simulink model "hall_effect_pos_vel_track"  (R2022a)
settings: Solver=FixedStepDiscrete  StartTime=0.0  StopTime=Inf  RelTol=1e-3  EnableMultiTasking=on
undefined symbols (not defined in the file or in its folder): Down, GPTRIP1SEL, GPTRIP2SEL, Hi, High, Impedance, TZ1, TZ2, Up, Z
libraries: c2802xlib x10, c2837xDlib x6, simulink x2, c2000lib x1
settings Model: SimulationMode=external  ExtModeTrigDuration=8  ExtModeArchiveFileName=pep  ExtModeArchiveDirName=C:\Users\adria\Desktop\motor_driver\logs  ExtModeAutoIncOneShot=on  Creator=adria  LastModifiedBy=EEED Stores 381
settings SolverCC: AlgebraicLoopSolver=TrustRegion
settings OptimizationCC: DefaultUnderspecifiedDataType=single  EnhancedBackFolding=on  PassReuseOutputArgsAs=Individual arguments  MaxStackSize=1024  OptimizeBlockOrder=speed  DifferentSizesBufferReuse=on  OptimizationCustomize=off  DenormalBehavior=FlushToZero  EfficientTunableParamExpr=on
settings DebuggingCC: MultiTaskDSMMsg=none  ParameterTunabilityLossMsg=error  UnconnectedInputMsg=warning  UnconnectedOutputMsg=warning  UnconnectedLineMsg=warning  SFMachineParentedDataDiag=warning
settings HardwareCC: ProdBitPerChar=16  ProdBitPerInt=16  ProdBitPerPointer=32  ProdBitPerSizeT=32  ProdBitPerPtrDiffT=32  ProdLargestAtomicInteger=Integer  ProdLargestAtomicFloat=None  ProdWordSize=16  ProdLongLongMode=on  ProdHWDeviceType=Texas Instruments->C2000
settings SFSimCC: MATLABDynamicMemAlloc=off
settings RTWCC: SystemTargetFile=ert.tlc  HardwareBoard=TI Delfino F28379D LaunchPad  TemplateMakefile=ert_default_tmf  Toolchain=Texas Instruments Code Composer Studio (C2000)  DLArmComputeVersion=19.05
settings CodeAppCC: ForceParamTrailComments=on  IgnoreCustomStorageClasses=off  OperatorAnnotations=on  SimulinkDataObjDesc=on  SFDataObjDesc=on  InsertBlockDesc=on
settings ERTTargetCC: CodeReplacementLibrary=TI C28x  ExtMode=on  ExtModeTransport=4  ExtModeStaticAlloc=on  ExtModeStaticAllocSize=10000  ExtModeMexFile=ext_xcp  ExtModeMexArgs='127.0.0.1' 0 17725  ExtModeIntrfLevel=Level2 - Open

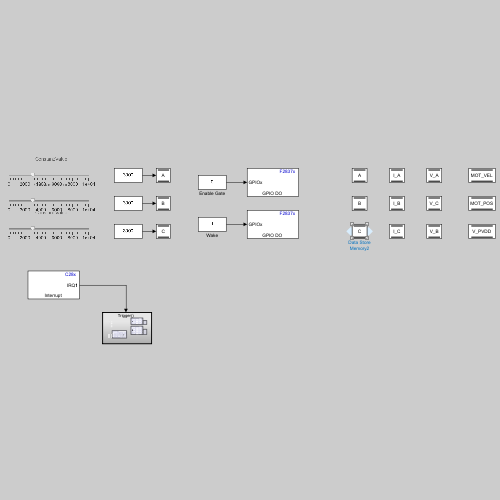
[thumbnail: Simulink's stored preview of the top-level diagram]
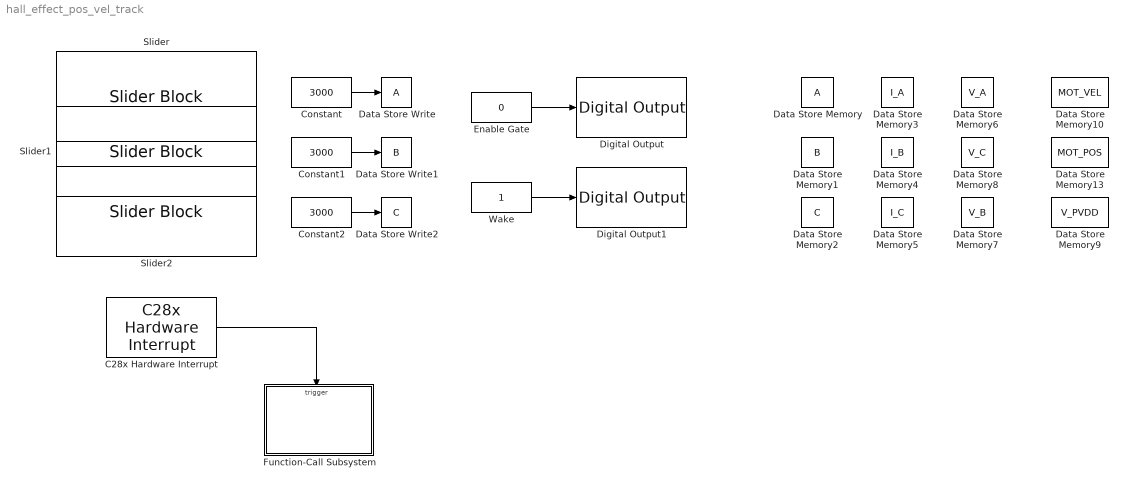
== system hall_effect_pos_vel_track ==
  C28x Hardware Interrupt : c2000lib/Scheduling/C28x Hardware Interrupt  irqnumbers=[1]  pienumbers=[1]  irqpriorities=[30]  irqpreempts=[0]  showinput=off  dspchiptype=C280X
      settings: SourceProductBaseCode=TIC2000
  Constant : Constant  Value=3000  OutDataTypeStr=uint32
  Constant1 : Constant  Value=3000  OutDataTypeStr=uint32
  Constant2 : Constant  Value=3000  OutDataTypeStr=uint32
  Data Store Memory : DataStoreMemory  ReadBeforeWriteMsg=warning  WriteAfterWriteMsg=warning  WriteAfterReadMsg=warning  ShowAdditionalParam=off  OutDataTypeStr=uint32
  Data Store Memory1 : DataStoreMemory  DataStoreName=B  ReadBeforeWriteMsg=warning  WriteAfterWriteMsg=warning  WriteAfterReadMsg=warning  ShowAdditionalParam=off  OutDataTypeStr=uint32
  Data Store Memory10 : DataStoreMemory  DataStoreName=MOT_VEL  ReadBeforeWriteMsg=warning  WriteAfterWriteMsg=warning  WriteAfterReadMsg=warning  ShowAdditionalParam=off  OutDataTypeStr=single
  Data Store Memory13 : DataStoreMemory  DataStoreName=MOT_POS  ReadBeforeWriteMsg=warning  WriteAfterWriteMsg=warning  WriteAfterReadMsg=warning  ShowAdditionalParam=off  OutDataTypeStr=single
  Data Store Memory2 : DataStoreMemory  DataStoreName=C  ReadBeforeWriteMsg=warning  WriteAfterWriteMsg=warning  WriteAfterReadMsg=warning  ShowAdditionalParam=off  OutDataTypeStr=uint32
  Data Store Memory3 : DataStoreMemory  DataStoreName=I_A  ReadBeforeWriteMsg=warning  WriteAfterWriteMsg=warning  WriteAfterReadMsg=warning  ShowAdditionalParam=off  OutDataTypeStr=single
  Data Store Memory4 : DataStoreMemory  DataStoreName=I_B  ReadBeforeWriteMsg=warning  WriteAfterWriteMsg=warning  WriteAfterReadMsg=warning  ShowAdditionalParam=off  OutDataTypeStr=single
  Data Store Memory5 : DataStoreMemory  DataStoreName=I_C  ReadBeforeWriteMsg=warning  WriteAfterWriteMsg=warning  WriteAfterReadMsg=warning  ShowAdditionalParam=off  OutDataTypeStr=single
  Data Store Memory6 : DataStoreMemory  DataStoreName=V_A  ReadBeforeWriteMsg=warning  WriteAfterWriteMsg=warning  WriteAfterReadMsg=warning  ShowAdditionalParam=off  OutDataTypeStr=single
  Data Store Memory7 : DataStoreMemory  DataStoreName=V_B  ReadBeforeWriteMsg=warning  WriteAfterWriteMsg=warning  WriteAfterReadMsg=warning  ShowAdditionalParam=off  OutDataTypeStr=single
  Data Store Memory8 : DataStoreMemory  DataStoreName=V_C  ReadBeforeWriteMsg=warning  WriteAfterWriteMsg=warning  WriteAfterReadMsg=warning  ShowAdditionalParam=off  OutDataTypeStr=single
  Data Store Memory9 : DataStoreMemory  DataStoreName=V_PVDD  ReadBeforeWriteMsg=warning  WriteAfterWriteMsg=warning  WriteAfterReadMsg=warning  ShowAdditionalParam=off  OutDataTypeStr=single
  Data Store Write : DataStoreWrite  IndexOptions=Index vector (dialog)  Indices=1  OutputSizes=1
  Data Store Write1 : DataStoreWrite  DataStoreName=B  IndexOptions=Index vector (dialog)  Indices=1  OutputSizes=1
  Data Store Write2 : DataStoreWrite  DataStoreName=C  IndexOptions=Index vector (dialog)  Indices=1  OutputSizes=1
  Digital Output : c2837xDlib/Digital Output  GPIO_Number=GPIO24~GPIO31  GPIO_Bit0=off  GPIO_BIT0_Toggle=off  GPIO_Bit1=off  GPIO_BIT1_Toggle=off  GPIO_Bit2=on  GPIO_BIT2_Toggle=off  GPIO_Bit3=off  GPIO_BIT3_Toggle=off  GPIO_Bit4=off  GPIO_BIT4_Toggle=off  GPIO_Bit5=off  GPIO_BIT5_Toggle=off  GPIO_Bit6=off  GPIO_BIT6_Toggle=off  GPIO_Bit7=off  GPIO_BIT7_Toggle=off
      settings: SourceProductBaseCode=TIC2000
  Digital Output1 : c2837xDlib/Digital Output  GPIO_Number=GPIO24~GPIO31  GPIO_Bit0=off  GPIO_BIT0_Toggle=off  GPIO_Bit1=off  GPIO_BIT1_Toggle=off  GPIO_Bit2=off  GPIO_BIT2_Toggle=off  GPIO_Bit3=on  GPIO_BIT3_Toggle=off  GPIO_Bit4=off  GPIO_BIT4_Toggle=off  GPIO_Bit5=off  GPIO_BIT5_Toggle=off  GPIO_Bit6=off  GPIO_BIT6_Toggle=off  GPIO_Bit7=off  GPIO_BIT7_Toggle=off
      settings: SourceProductBaseCode=TIC2000
  Enable Gate : Constant  Value=0  OutDataTypeStr=uint32
  Function-Call Subsystem : Subsystem  TreatAsAtomicUnit=on
  Slider : SliderBlock  ScaleMax=10e3
  Slider1 : SliderBlock  ScaleMax=10e3
  Slider2 : SliderBlock  ScaleMax=10e3
  Wake : Constant  OutDataTypeStr=uint32
  wires:
  Enable Gate/1 -> Digital Output/1
  C28x Hardware Interrupt/1 -> Function-Call Subsystem/Trigger
  Constant/1 -> Data Store Write/1
  Constant1/1 -> Data Store Write1/1
  Constant2/1 -> Data Store Write2/1
  Wake/1 -> Digital Output1/1

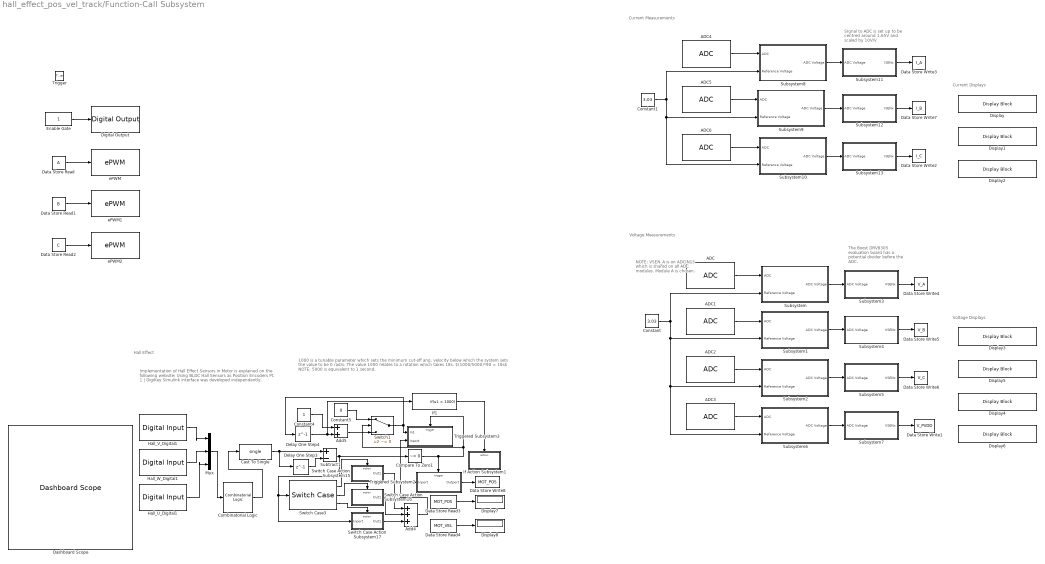
== system hall_effect_pos_vel_track/Function-Call Subsystem ==
  note: Voltage Displays
  note: Current Displays
  note: Current Measurements
  note: Voltage Measurements
  note: NOTE: VSEN_A is on ADCIN15 which is shared on all ADC modules. Module A is chosen.
  note: The Boost DRV8305 evaluation board has a potential divider before the ADC.
  note: SIgnal to ADC is set up to be centred around 1.65V and scaled by 10V/V
  note: 1000 is a tunable parameter which sets the minimum cut-off ang. velocity below which the system sets the value to be 0 rad/s. The value 1000 relates to a rotation which takes 18s.
      | $(1000/5000)*90 = 18s$
      | NOTE: 5000 is equivalent to 1 second.
  note: Hall Effect
  note: Implementation of Hall Effect Sensors in Motor is explained on the following website:
      | Using BLDC Hall Sensors as Position Encoders Pt. 1 | DigiKey
      |
      | Simulink interface was developed independently.
  Trigger : TriggerPort  TriggerType=function-call  VariantControl=Variant  PortDimensions=1
  ADC : c2802xlib/ADC  blkParamProc=C2000_Type4  ADCModule=A  samplingMode=Single sample mode  ADCResolution=12-bit (Single-ended input)  useSOC1=SOC1  useSOC2=SOC0_SOC1  SOCAcquisitionWindow=63  SOCTriggerSource=ePWM4_ADCSOCA  SOCInterruptTrigger=No ADCINT  Ts=-1  dType=uint16  postInterrupt=off  interruptSel=ADCINT2  ADCINTContinuous=off  endma=off  chdma=1  conv1=ADCINA0  conv2=ADCINA0 and ADCINB0  conv1_Type4=ADCIN15  conv2_Type4=ADCIN0 and ADCIN1
      settings: SourceProductName=Embedded Coder Support Package for Texas Instruments C2000 Processors
  ADC1 : c2802xlib/ADC  blkParamProc=C2000_Type4  ADCModule=C  samplingMode=Single sample mode  ADCResolution=12-bit (Single-ended input)  useSOC1=SOC1  useSOC2=SOC0_SOC1  SOCAcquisitionWindow=63  SOCTriggerSource=ePWM4_ADCSOCA  SOCInterruptTrigger=No ADCINT  Ts=-1  dType=uint16  postInterrupt=off  interruptSel=ADCINT1  ADCINTContinuous=off  endma=off  chdma=1  conv1=ADCINA0  conv2=ADCINA0 and ADCINB0  conv1_Type4=ADCIN5  conv2_Type4=ADCIN0 and ADCIN1
      settings: SourceProductName=Embedded Coder Support Package for Texas Instruments C2000 Processors
  ADC2 : c2802xlib/ADC  blkParamProc=C2000_Type4  ADCModule=B  samplingMode=Single sample mode  ADCResolution=12-bit (Single-ended input)  useSOC1=SOC1  useSOC2=SOC0_SOC1  SOCAcquisitionWindow=63  SOCTriggerSource=ePWM4_ADCSOCA  SOCInterruptTrigger=No ADCINT  Ts=-1  dType=uint16  postInterrupt=off  interruptSel=ADCINT1  ADCINTContinuous=off  endma=off  chdma=1  conv1=ADCINA0  conv2=ADCINA0 and ADCINB0  conv1_Type4=ADCIN5  conv2_Type4=ADCIN0 and ADCIN1
      settings: SourceProductName=Embedded Coder Support Package for Texas Instruments C2000 Processors
  ADC3 : c2802xlib/ADC  blkParamProc=C2000_Type4  ADCModule=A  samplingMode=Single sample mode  ADCResolution=12-bit (Single-ended input)  useSOC1=SOC2  useSOC2=SOC0_SOC1  SOCAcquisitionWindow=63  SOCTriggerSource=ePWM4_ADCSOCA  SOCInterruptTrigger=No ADCINT  Ts=-1  dType=uint16  postInterrupt=on  interruptSel=ADCINT1  ADCINTContinuous=off  endma=off  chdma=1  conv1=ADCINA0  conv2=ADCINA0 and ADCINB0  conv1_Type4=ADCIN5  conv2_Type4=ADCIN0 and ADCIN1
      settings: SourceProductName=Embedded Coder Support Package for Texas Instruments C2000 Processors
  ADC4 : c2802xlib/ADC  blkParamProc=C2000_Type4  ADCModule=C  samplingMode=Single sample mode  ADCResolution=12-bit (Single-ended input)  useSOC1=SOC0  useSOC2=SOC0_SOC1  SOCAcquisitionWindow=63  SOCTriggerSource=ePWM4_ADCSOCA  SOCInterruptTrigger=No ADCINT  Ts=-1  dType=uint16  postInterrupt=off  interruptSel=ADCINT2  ADCINTContinuous=off  endma=off  chdma=1  conv1=ADCINA0  conv2=ADCINA0 and ADCINB0  conv1_Type4=ADCIN4  conv2_Type4=ADCIN0 and ADCIN1
      settings: SourceProductName=Embedded Coder Support Package for Texas Instruments C2000 Processors
  ADC5 : c2802xlib/ADC  blkParamProc=C2000_Type4  ADCModule=B  samplingMode=Single sample mode  ADCResolution=12-bit (Single-ended input)  useSOC1=SOC0  useSOC2=SOC0_SOC1  SOCAcquisitionWindow=63  SOCTriggerSource=ePWM4_ADCSOCA  SOCInterruptTrigger=No ADCINT  Ts=-1  dType=uint16  postInterrupt=off  interruptSel=ADCINT2  ADCINTContinuous=off  endma=off  chdma=1  conv1=ADCINA0  conv2=ADCINA0 and ADCINB0  conv1_Type4=ADCIN4  conv2_Type4=ADCIN0 and ADCIN1
      settings: SourceProductName=Embedded Coder Support Package for Texas Instruments C2000 Processors
  ADC6 : c2802xlib/ADC  blkParamProc=C2000_Type4  ADCModule=A  samplingMode=Single sample mode  ADCResolution=12-bit (Single-ended input)  useSOC1=SOC0  useSOC2=SOC0_SOC1  SOCAcquisitionWindow=63  SOCTriggerSource=ePWM4_ADCSOCA  SOCInterruptTrigger=No ADCINT  Ts=-1  dType=uint16  postInterrupt=off  interruptSel=ADCINT1  ADCINTContinuous=on  endma=off  chdma=1  conv1=ADCINA0  conv2=ADCINA0 and ADCINB0  conv1_Type4=ADCIN4  conv2_Type4=ADCIN0 and ADCIN1
      settings: SourceProductName=Embedded Coder Support Package for Texas Instruments C2000 Processors
  Add4 : Sum  Inputs=+++  AccumDataTypeStr=single
  Add5 : Sum
  Cast To Single : DataTypeConversion  OutDataTypeStr=single  SaturateOnIntegerOverflow=off  RndMeth=Floor
  Combinatorial Logic : CombinatorialLogic  TruthTable=[0;1;3;2;5;6;4;7]
  Compare To Zero1 : simulink/Logic and Bit Operations/Compare To Zero  relop=~=  OutDataTypeStr=boolean
  Constant : Constant  Value=3.03  OutDataTypeStr=single
  Constant1 : Constant  Value=3.03  OutDataTypeStr=single
  Constant4 : Constant  OutDataTypeStr=single
  Constant5 : Constant  Value=0  OutDataTypeStr=single
  Dashboard Scope : DashboardScope  TimeSpan=5  Ymin=0  Ymax=7  ScaleAtStop=off
  Data Store Read : DataStoreRead  IndexOptions=Index vector (dialog)  Indices=1  OutputSizes=1
  Data Store Read1 : DataStoreRead  DataStoreName=B  IndexOptions=Index vector (dialog)  Indices=1  OutputSizes=1
  Data Store Read2 : DataStoreRead  DataStoreName=C  IndexOptions=Index vector (dialog)  Indices=1  OutputSizes=1
  Data Store Read3 : DataStoreRead  DataStoreName=MOT_POS  IndexOptions=Index vector (dialog)  Indices=1  OutputSizes=1
  Data Store Read4 : DataStoreRead  DataStoreName=MOT_VEL  IndexOptions=Index vector (dialog)  Indices=1  OutputSizes=1
  Data Store Write1 : DataStoreWrite  DataStoreName=V_PVDD  IndexOptions=Index vector (dialog)  Indices=1  OutputSizes=1
  Data Store Write2 : DataStoreWrite  DataStoreName=I_C  IndexOptions=Index vector (dialog)  Indices=1  OutputSizes=1
  Data Store Write3 : DataStoreWrite  DataStoreName=I_A  IndexOptions=Index vector (dialog)  Indices=1  OutputSizes=1
  Data Store Write4 : DataStoreWrite  DataStoreName=V_A  IndexOptions=Index vector (dialog)  Indices=1  OutputSizes=1
  Data Store Write5 : DataStoreWrite  DataStoreName=V_B  IndexOptions=Index vector (dialog)  Indices=1  OutputSizes=1
  Data Store Write6 : DataStoreWrite  DataStoreName=V_C  IndexOptions=Index vector (dialog)  Indices=1  OutputSizes=1
  Data Store Write7 : DataStoreWrite  DataStoreName=I_B  IndexOptions=Index vector (dialog)  Indices=1  OutputSizes=1
  Data Store Write8 : DataStoreWrite  DataStoreName=MOT_POS  IndexOptions=Index vector (dialog)  Indices=1  OutputSizes=1
  Delay One Step3 : Delay  DelayLength=1
  Delay One Step4 : Delay  DelayLength=1
  Digital Output : c2837xDlib/Digital Output  GPIO_Number=GPIO48~GPIO55  GPIO_Bit0=off  GPIO_BIT0_Toggle=off  GPIO_Bit1=off  GPIO_BIT1_Toggle=off  GPIO_Bit2=off  GPIO_BIT2_Toggle=off  GPIO_Bit3=off  GPIO_BIT3_Toggle=off  GPIO_Bit4=on  GPIO_BIT4_Toggle=on  GPIO_Bit5=off  GPIO_BIT5_Toggle=off  GPIO_Bit6=off  GPIO_BIT6_Toggle=off  GPIO_Bit7=off  GPIO_BIT7_Toggle=off
      settings: SourceProductBaseCode=TIC2000
  Display{,1..6} (7 alike) : DisplayBlock  LabelPosition=Hide  Transparency=1
  Display7 : Display
  Display8 : Display
  Enable Gate : Constant  OutDataTypeStr=uint32
  Hall_U_Digital1 : c2837xDlib/Digital Input  GPIO_Number=GPIO120~GPIO127  GPIO_Bit0=off  GPIO_Bit1=off  GPIO_Bit2=off  GPIO_Bit3=off  GPIO_Bit4=on  GPIO_Bit5=off  GPIO_Bit6=off  GPIO_Bit7=off  sampleTime=-1  dataType=auto  GPIO_Bit0_Qualification=Sync to SYSCLKOUT  GPIO_Bit1_Qualification=Sync to SYSCLKOUT  GPIO_Bit2_Qualification=Sync to SYSCLKOUT  GPIO_Bit3_Qualification=Sync to SYSCLKOUT  GPIO_Bit4_Qualification=Sync to SYSCLKOUT  GPIO_Bit5_Qualification=Sync to SYSCLKOUT  GPIO_Bit6_Qualification=Sync to SYSCLKOUT  GPIO_Bit7_Qualification=Sync to SYSCLKOUT  Qualification_Period=-1
      settings: SourceProductBaseCode=TIC2000
  Hall_V_Digital1 : c2837xDlib/Digital Input  GPIO_Number=GPIO24~GPIO31  GPIO_Bit0=off  GPIO_Bit1=off  GPIO_Bit2=off  GPIO_Bit3=off  GPIO_Bit4=off  GPIO_Bit5=on  GPIO_Bit6=off  GPIO_Bit7=off  sampleTime=-1  dataType=auto  GPIO_Bit0_Qualification=Sync to SYSCLKOUT  GPIO_Bit1_Qualification=Sync to SYSCLKOUT  GPIO_Bit2_Qualification=Sync to SYSCLKOUT  GPIO_Bit3_Qualification=Sync to SYSCLKOUT  GPIO_Bit4_Qualification=Sync to SYSCLKOUT  GPIO_Bit5_Qualification=Sync to SYSCLKOUT  GPIO_Bit6_Qualification=Sync to SYSCLKOUT  GPIO_Bit7_Qualification=Sync to SYSCLKOUT  Qualification_Period=-1
      settings: SourceProductBaseCode=TIC2000
  Hall_W_Digital1 : c2837xDlib/Digital Input  GPIO_Number=GPIO120~GPIO127  GPIO_Bit0=off  GPIO_Bit1=off  GPIO_Bit2=off  GPIO_Bit3=off  GPIO_Bit4=off  GPIO_Bit5=on  GPIO_Bit6=off  GPIO_Bit7=off  sampleTime=-1  dataType=auto  GPIO_Bit0_Qualification=Sync to SYSCLKOUT  GPIO_Bit1_Qualification=Sync to SYSCLKOUT  GPIO_Bit2_Qualification=Sync to SYSCLKOUT  GPIO_Bit3_Qualification=Sync to SYSCLKOUT  GPIO_Bit4_Qualification=Sync to SYSCLKOUT  GPIO_Bit5_Qualification=Sync to SYSCLKOUT  GPIO_Bit6_Qualification=Sync to SYSCLKOUT  GPIO_Bit7_Qualification=Sync to SYSCLKOUT  Qualification_Period=-1
      settings: SourceProductBaseCode=TIC2000
  If Action Subsystem1 : Subsystem  TreatAsAtomicUnit=on
  If1 : If  IfExpression=u1 > 1000  ShowElse=off
  Mux : Mux  Inputs=3
  Subsystem : Subsystem
  Subsystem1 : Subsystem
  Subsystem10 : Subsystem
  Subsystem11 : Subsystem
  Subsystem12 : Subsystem
  Subsystem13 : Subsystem
  Subsystem2 : Subsystem
  Subsystem3 : Subsystem
  Subsystem4 : Subsystem
  Subsystem5 : Subsystem
  Subsystem6 : Subsystem
  Subsystem7 : Subsystem
  Subsystem8 : Subsystem
  Subsystem9 : Subsystem
  Subtract1 : Sum  Inputs=+-
  Switch Case Action Subsystem15 : Subsystem  TreatAsAtomicUnit=on
  Switch Case Action Subsystem16 : Subsystem  TreatAsAtomicUnit=on
  Switch Case Action Subsystem17 : Subsystem  TreatAsAtomicUnit=on
  Switch Case3 : SwitchCase  CaseConditions={-5,5}
  Switch1 : Switch  Criteria=u2 ~= 0  SaturateOnIntegerOverflow=off  InputSameDT=off
  Triggered Subsystem2 : Subsystem  TreatAsAtomicUnit=on
  Triggered Subsystem3 : Subsystem  TreatAsAtomicUnit=on
  ePWM : c2802xlib/ePWM  PwmType=C2000_Type4  useModule=ePWM4  ePWMxLINKTBPRD=Not Linked  periodUnits=Seconds  timerSource=Specify via dialog  timerPeriod_clk=64000  timerPeriod_sec=1/10e3  tbshadow=Counter equals to zero  countingMode=Up-Down  phaseActiveEnable=Disable  phaseDirection=Count down after sync  phaseActive=0  synchronizationEnable=off  dcaevt1Sync=off  dcbevt1Sync=off  synchronizationOption=Counter equals to zero (CTR=Zero)  perSynchronizationOption=Counter equals to period (CTR=PRD)  clockPrescale=1  HSclockPrescale=1  enswap=off  ePWMxAStatus=on  ePWMxAactionLogic1=Set  ePWMxAactionLogic2=Clear  ePWMxAactionLogic3=Clear  ePWMxAactionLogic4=Set  ePWMxAactionLogic5=Do nothing  ePWMxAactionLogic6=Do nothing  ePWMxACSFenable=off  ePWMxACSFvalue=Forcing disable  ePWMxASFreload=Zero  ePWMxBStatus=on  ePWMxBactionLogic1=Clear  ePWMxBactionLogic2=Set  ePWMxBactionLogic3=Set  ePWMxBactionLogic4=Clear  ePWMxBactionLogic5=Do nothing  ePWMxBactionLogic6=Do nothing  ePWMxBCSFenable=off  ePWMxBCSFvalue=Forcing disable  ePWMxBSFreload=Zero  ePWNxBOutWay=off  ePWMxLINKCMPA=Not Linked  CMPAUnits=Clock cycles  CMPASource=Input port  CMPAValue_per=50  CMPAValue_clk=32000  enCMPAshadow=Counter equals to zero (CTR=Zero)  ePWMxLINKCMPB=Not Linked  CMPBUnits=Clock cycles  CMPBSource=Specify via dialog  CMPBValue_per=50  CMPBValue_clk=32000  enCMPBshadow=Counter equals to zero (CTR=Zero)  ePWMxLINKCMPC=Not Linked  CMPCUnits=Clock cycles  CMPCSource=Specify via dialog  CMPCValue_per=50  CMPCValue_clk=32000  enCMPCshadow=Counter equals to zero (CTR=Zero)  ePWMxLINKCMPD=Not Linked  CMPDUnits=Clock cycles  CMPDSource=Specify via dialog  CMPDValue_per=50  CMPDValue_clk=32000  enCMPDshadow=Counter equals to zero (CTR=Zero)  enableDBePWMxA=on  enableDBePWMxB=on  enhalfcycle=off  DBpolarity=Active high complementary (AHC)  DBedgeDelay=Positive  DBSource_ePWMxA=ePWMxA  DBSource_ePWMxB=ePWMxA  DBPeriodUnits=Clock cycles  DBperiodSource=Specify via dialog  REDperiod=10  FEDperiod=10  REDperiod_sec=0  FEDperiod_sec=0  LoadModeDBRED=Immediate without using shadow  LoadModeDBFED=Immediate without using shadow  adcstartModuleA=on  adcrequestEventA=First event  adcstartEventA=Digital Compare Module A Event 1 start of conversion (DCAEVT1.soc)  adcstartEventA_type2=Counter equals to zero (CTR=Zero)  adcstartModuleB=off  adcrequestEventB=First event  adcstartEventB=Counter equals to zero (CTR=Zero)  adcstartEventB_type2=Counter equals to zero (CTR=Zero)  intEn=off  intPrd=First event  intSel=Counter equals to zero (CTR=Zero)  intSel_type2=Counter equals to zero (CTR=Zero)  hrpe=off  enHRPWM=off  HRPWM_LoadMode=Counter equals to period (CTR=PRD)  HRPWM_CTLMode=Duty or Period control mode  HRPWM_EDGMode=Both edge  hrpeb=off  enHRPWMB=off  HRPWM_LoadModeB=Counter equals to zero (CTR=ZERO)  HRPWM_CTLModeB=Duty or Period control mode  HRPWM_EDGModeB=Both edge  enHRDBRED=off  enHRDBFED=off  enSFO=on  enautoconv=on  chopperEnable=off  chopperFrequency=1  chopperFirstwidth=1  chopperDuty=12.5%  tripZonesource=Specify via dialog  tzselOSHT1=off  tzselOSHT2=off  tzselOSHT3=off  tzselOSHDCAEV1=off  tzselOSHDCBEV1=off  tzselCBC1=off  tzselCBC2=off  tzselCBC3=off  tzselCBCDCAEV2=off  tzselCBCDCBEV2=off  tzselOSHT4=off  tzselOSHT5=off  tzselOSHT6=off  tzselCBC4=off  tzselCBC5=off  tzselCBC6=off  enTzOstIntr=off  enTzCbcIntr=off  enTzDCAEVT1Intr=off  enTzDCAEVT2Intr=off  enTzDCBEVT1Intr=off  enTzDCBEVT2Intr=off  ePWMxAforced=Hi-Z(High-Impedance)  ePWMxBforced=Hi-Z(High-Impedance)  DCAEVT1forced=No action  DCBEVT1forced=No action  DCAEVT2forced=No action  DCBEVT2forced=No action  dcah=Trip Zone 1 input (TZ1)  dcal=Trip Zone 2 input (TZ2)  dcbh=Trip Zone 1 input (TZ1)  dcbl=Trip Zone 2 input (TZ2)  dcah_type2=GPTRIP1SEL/(TZ1)  dcal_type2=GPTRIP2SEL/(TZ2)  dcbh_type2=GPTRIP1SEL/(TZ1)  dcbl_type2=GPTRIP2SEL/(TZ2)  gendcaevt1=Event disabled  gendcaevt2=Event disabled  gendcbevt1=Event disabled  gendcbevt2=Event disabled  dcaevt1src=DCAEVT1 with sync  dcaevt2src=DCAEVT2 with sync  dcbevt1src=DCBEVT1 with sync  dcbevt2src=DCBEVT2 with sync  pulsesel=Counter equals to zero (CTR=Zero)  blankinv=off  blankoffset=0  blankwidth=0  evsrcsel=Filtered version of DCAEVT1 (DCAEVT1FILT)  encape=off
      settings: SourceProductName=Embedded Coder Support Package for Texas Instruments C2000 Processors
  ePWM1 : c2802xlib/ePWM  PwmType=C2000_Type4  useModule=ePWM5  ePWMxLINKTBPRD=Not Linked  periodUnits=Seconds  timerSource=Specify via dialog  timerPeriod_clk=64000  timerPeriod_sec=1/10e3  tbshadow=Counter equals to zero  countingMode=Up-Down  phaseActiveEnable=Set counter to phase value specified via dialog  phaseDirection=Count down after sync  phaseActive=0  synchronizationEnable=off  dcaevt1Sync=off  dcbevt1Sync=off  synchronizationOption=Pass through (EPWMxSYNCI or SWFSYNC)  perSynchronizationOption=Counter equals to period (CTR=PRD)  clockPrescale=1  HSclockPrescale=1  enswap=off  ePWMxAStatus=on  ePWMxAactionLogic1=Set  ePWMxAactionLogic2=Clear  ePWMxAactionLogic3=Clear  ePWMxAactionLogic4=Set  ePWMxAactionLogic5=Do nothing  ePWMxAactionLogic6=Do nothing  ePWMxACSFenable=off  ePWMxACSFvalue=Forcing disable  ePWMxASFreload=Zero  ePWMxBStatus=on  ePWMxBactionLogic1=Clear  ePWMxBactionLogic2=Set  ePWMxBactionLogic3=Set  ePWMxBactionLogic4=Clear  ePWMxBactionLogic5=Do nothing  ePWMxBactionLogic6=Do nothing  ePWMxBCSFenable=off  ePWMxBCSFvalue=Forcing disable  ePWMxBSFreload=Zero  ePWNxBOutWay=off  ePWMxLINKCMPA=Not Linked  CMPAUnits=Clock cycles  CMPASource=Input port  CMPAValue_per=50  CMPAValue_clk=32000  enCMPAshadow=Counter equals to zero (CTR=Zero)  ePWMxLINKCMPB=Not Linked  CMPBUnits=Clock cycles  CMPBSource=Specify via dialog  CMPBValue_per=50  CMPBValue_clk=32000  enCMPBshadow=Counter equals to zero (CTR=Zero)  ePWMxLINKCMPC=Not Linked  CMPCUnits=Clock cycles  CMPCSource=Specify via dialog  CMPCValue_per=50  CMPCValue_clk=32000  enCMPCshadow=Counter equals to zero (CTR=Zero)  ePWMxLINKCMPD=Not Linked  CMPDUnits=Clock cycles  CMPDSource=Specify via dialog  CMPDValue_per=50  CMPDValue_clk=32000  enCMPDshadow=Counter equals to zero (CTR=Zero)  enableDBePWMxA=on  enableDBePWMxB=on  enhalfcycle=off  DBpolarity=Active high complementary (AHC)  DBedgeDelay=Positive  DBSource_ePWMxA=ePWMxA  DBSource_ePWMxB=ePWMxA  DBPeriodUnits=Clock cycles  DBperiodSource=Specify via dialog  REDperiod=10  FEDperiod=10  REDperiod_sec=0  FEDperiod_sec=0  LoadModeDBRED=Immediate without using shadow  LoadModeDBFED=Immediate without using shadow  adcstartModuleA=off  adcrequestEventA=First event  adcstartEventA=Digital Compare Module A Event 1 start of conversion (DCAEVT1.soc)  adcstartEventA_type2=Digital Compare Module A Event 1 start of conversion (DCAEVT1.soc)  adcstartModuleB=off  adcrequestEventB=First event  adcstartEventB=Counter equals to zero (CTR=Zero)  adcstartEventB_type2=Counter equals to zero (CTR=Zero)  intEn=off  intPrd=First event  intSel=Counter equals to zero (CTR=Zero)  intSel_type2=Counter equals to zero (CTR=Zero)  hrpe=off  enHRPWM=off  HRPWM_LoadMode=Counter equals to period (CTR=PRD)  HRPWM_CTLMode=Duty or Period control mode  HRPWM_EDGMode=Both edge  hrpeb=off  enHRPWMB=off  HRPWM_LoadModeB=Counter equals to zero (CTR=ZERO)  HRPWM_CTLModeB=Duty or Period control mode  HRPWM_EDGModeB=Both edge  enHRDBRED=off  enHRDBFED=off  enSFO=on  enautoconv=on  chopperEnable=off  chopperFrequency=1  chopperFirstwidth=1  chopperDuty=12.5%  tripZonesource=Specify via dialog  tzselOSHT1=off  tzselOSHT2=off  tzselOSHT3=off  tzselOSHDCAEV1=off  tzselOSHDCBEV1=off  tzselCBC1=off  tzselCBC2=off  tzselCBC3=off  tzselCBCDCAEV2=off  tzselCBCDCBEV2=off  tzselOSHT4=off  tzselOSHT5=off  tzselOSHT6=off  tzselCBC4=off  tzselCBC5=off  tzselCBC6=off  enTzOstIntr=off  enTzCbcIntr=off  enTzDCAEVT1Intr=off  enTzDCAEVT2Intr=off  enTzDCBEVT1Intr=off  enTzDCBEVT2Intr=off  ePWMxAforced=No action  ePWMxBforced=No action  DCAEVT1forced=No action  DCBEVT1forced=No action  DCAEVT2forced=No action  DCBEVT2forced=No action  dcah=Trip Zone 1 input (TZ1)  dcal=Trip Zone 2 input (TZ2)  dcbh=Trip Zone 1 input (TZ1)  dcbl=Trip Zone 2 input (TZ2)  dcah_type2=GPTRIP1SEL/(TZ1)  dcal_type2=GPTRIP2SEL/(TZ2)  dcbh_type2=GPTRIP1SEL/(TZ1)  dcbl_type2=GPTRIP2SEL/(TZ2)  gendcaevt1=Event disabled  gendcaevt2=Event disabled  gendcbevt1=Event disabled  gendcbevt2=Event disabled  dcaevt1src=DCAEVT1 with sync  dcaevt2src=DCAEVT2 with sync  dcbevt1src=DCBEVT1 with sync  dcbevt2src=DCBEVT2 with sync  pulsesel=Counter equals to zero (CTR=Zero)  blankinv=off  blankoffset=0  blankwidth=0  evsrcsel=Filtered version of DCAEVT1 (DCAEVT1FILT)  encape=off
      settings: SourceProductName=Embedded Coder Support Package for Texas Instruments C2000 Processors
  ePWM2 : c2802xlib/ePWM  PwmType=C2000_Type4  useModule=ePWM6  ePWMxLINKTBPRD=Not Linked  periodUnits=Seconds  timerSource=Specify via dialog  timerPeriod_clk=64000  timerPeriod_sec=1/10e3  tbshadow=Counter equals to zero  countingMode=Up-Down  phaseActiveEnable=Set counter to phase value specified via dialog  phaseDirection=Count down after sync  phaseActive=0  synchronizationEnable=off  dcaevt1Sync=off  dcbevt1Sync=off  synchronizationOption=Disable  perSynchronizationOption=Counter equals to period (CTR=PRD)  clockPrescale=1  HSclockPrescale=1  enswap=off  ePWMxAStatus=on  ePWMxAactionLogic1=Set  ePWMxAactionLogic2=Clear  ePWMxAactionLogic3=Clear  ePWMxAactionLogic4=Set  ePWMxAactionLogic5=Do nothing  ePWMxAactionLogic6=Do nothing  ePWMxACSFenable=off  ePWMxACSFvalue=Forcing disable  ePWMxASFreload=Zero  ePWMxBStatus=on  ePWMxBactionLogic1=Clear  ePWMxBactionLogic2=Set  ePWMxBactionLogic3=Set  ePWMxBactionLogic4=Clear  ePWMxBactionLogic5=Do nothing  ePWMxBactionLogic6=Do nothing  ePWMxBCSFenable=off  ePWMxBCSFvalue=Forcing disable  ePWMxBSFreload=Zero  ePWNxBOutWay=off  ePWMxLINKCMPA=Not Linked  CMPAUnits=Clock cycles  CMPASource=Input port  CMPAValue_per=50  CMPAValue_clk=32000  enCMPAshadow=Counter equals to zero (CTR=Zero)  ePWMxLINKCMPB=Not Linked  CMPBUnits=Clock cycles  CMPBSource=Specify via dialog  CMPBValue_per=50  CMPBValue_clk=32000  enCMPBshadow=Counter equals to zero (CTR=Zero)  ePWMxLINKCMPC=Not Linked  CMPCUnits=Clock cycles  CMPCSource=Specify via dialog  CMPCValue_per=50  CMPCValue_clk=32000  enCMPCshadow=Counter equals to zero (CTR=Zero)  ePWMxLINKCMPD=Not Linked  CMPDUnits=Clock cycles  CMPDSource=Specify via dialog  CMPDValue_per=50  CMPDValue_clk=32000  enCMPDshadow=Counter equals to zero (CTR=Zero)  enableDBePWMxA=on  enableDBePWMxB=on  enhalfcycle=off  DBpolarity=Active high complementary (AHC)  DBedgeDelay=Positive  DBSource_ePWMxA=ePWMxA  DBSource_ePWMxB=ePWMxA  DBPeriodUnits=Clock cycles  DBperiodSource=Specify via dialog  REDperiod=10  FEDperiod=10  REDperiod_sec=0  FEDperiod_sec=0  LoadModeDBRED=Immediate without using shadow  LoadModeDBFED=Immediate without using shadow  adcstartModuleA=off  adcrequestEventA=First event  adcstartEventA=Digital Compare Module A Event 1 start of conversion (DCAEVT1.soc)  adcstartEventA_type2=Digital Compare Module A Event 1 start of conversion (DCAEVT1.soc)  adcstartModuleB=off  adcrequestEventB=First event  adcstartEventB=Counter equals to zero (CTR=Zero)  adcstartEventB_type2=Counter equals to zero (CTR=Zero)  intEn=off  intPrd=First event  intSel=Counter equals to zero (CTR=Zero)  intSel_type2=Counter equals to zero (CTR=Zero)  hrpe=off  enHRPWM=off  HRPWM_LoadMode=Counter equals to period (CTR=PRD)  HRPWM_CTLMode=Duty or Period control mode  HRPWM_EDGMode=Both edge  hrpeb=off  enHRPWMB=off  HRPWM_LoadModeB=Counter equals to zero (CTR=ZERO)  HRPWM_CTLModeB=Duty or Period control mode  HRPWM_EDGModeB=Both edge  enHRDBRED=off  enHRDBFED=off  enSFO=on  enautoconv=on  chopperEnable=off  chopperFrequency=1  chopperFirstwidth=1  chopperDuty=12.5%  tripZonesource=Specify via dialog  tzselOSHT1=off  tzselOSHT2=off  tzselOSHT3=off  tzselOSHDCAEV1=off  tzselOSHDCBEV1=off  tzselCBC1=off  tzselCBC2=off  tzselCBC3=off  tzselCBCDCAEV2=off  tzselCBCDCBEV2=off  tzselOSHT4=off  tzselOSHT5=off  tzselOSHT6=off  tzselCBC4=off  tzselCBC5=off  tzselCBC6=off  enTzOstIntr=off  enTzCbcIntr=off  enTzDCAEVT1Intr=off  enTzDCAEVT2Intr=off  enTzDCBEVT1Intr=off  enTzDCBEVT2Intr=off  ePWMxAforced=No action  ePWMxBforced=No action  DCAEVT1forced=No action  DCBEVT1forced=No action  DCAEVT2forced=No action  DCBEVT2forced=No action  dcah=Trip Zone 1 input (TZ1)  dcal=Trip Zone 2 input (TZ2)  dcbh=Trip Zone 1 input (TZ1)  dcbl=Trip Zone 2 input (TZ2)  dcah_type2=GPTRIP1SEL/(TZ1)  dcal_type2=GPTRIP2SEL/(TZ2)  dcbh_type2=GPTRIP1SEL/(TZ1)  dcbl_type2=GPTRIP2SEL/(TZ2)  gendcaevt1=Event disabled  gendcaevt2=Event disabled  gendcbevt1=Event disabled  gendcbevt2=Event disabled  dcaevt1src=DCAEVT1 with sync  dcaevt2src=DCAEVT2 with sync  dcbevt1src=DCBEVT1 with sync  dcbevt2src=DCBEVT2 with sync  pulsesel=Counter equals to zero (CTR=Zero)  blankinv=off  blankoffset=0  blankwidth=0  evsrcsel=Filtered version of DCAEVT1 (DCAEVT1FILT)  encape=off
      settings: SourceProductName=Embedded Coder Support Package for Texas Instruments C2000 Processors
  wires:
  Enable Gate/1 -> Digital Output/1
  Data Store Read/1 -> ePWM/1
  Data Store Read1/1 -> ePWM1/1
  Data Store Read2/1 -> ePWM2/1
  ADC3/1 -> Subsystem6/1(ADC)
  Subsystem3/1(VSENx) -> Data Store Write4/1
  Constant/1 -> Subsystem/2(Reference Voltage), Subsystem1/2(Reference Voltage), Subsystem6/2(Reference Voltage), Subsystem2/2(Reference Voltage)
  Subsystem7/1(VSENx) -> Data Store Write1/1
  Subsystem6/1(ADC Voltage) -> Subsystem7/1(ADC Voltage)
  ADC2/1 -> Subsystem2/1(ADC)
  ADC1/1 -> Subsystem1/1(ADC)
  ADC/1 -> Subsystem/1(ADC)
  Subsystem1/1(ADC Voltage) -> Subsystem4/1(ADC Voltage)
  Subsystem5/1(VSENx) -> Data Store Write6/1
  Subsystem2/1(ADC Voltage) -> Subsystem5/1(ADC Voltage)
  Subsystem4/1(VSENx) -> Data Store Write5/1
  Subsystem/1(ADC Voltage) -> Subsystem3/1(ADC Voltage)
  Subsystem13/1(ISENx) -> Data Store Write2/1
  Subsystem12/1(ISENx) -> Data Store Write7/1
  Subsystem9/1(ADC Voltage) -> Subsystem12/1(ADC Voltage)
  Subsystem11/1(ISENx) -> Data Store Write3/1
  Subsystem8/1(ADC Voltage) -> Subsystem11/1(ADC Voltage)
  ADC4/1 -> Subsystem8/1(ADC)
  ADC5/1 -> Subsystem9/1(ADC)
  Constant1/1 -> Subsystem8/2(Reference Voltage), Subsystem10/2(Reference Voltage), Subsystem9/2(Reference Voltage)
  ADC6/1 -> Subsystem10/1(ADC)
  Subsystem10/1(ADC Voltage) -> Subsystem13/1(ADC Voltage)
  If1/1 -> If Action Subsystem1/Action
  Switch Case3/1 -> Switch Case Action Subsystem15/Action
  Data Store Read4/1 -> Display8/1
  Triggered Subsystem2/1(Outport) -> Data Store Write8/1
  Delay One Step3/1 -> Subtract1/2
  Constant4/1 -> Add5/1
  Constant5/1 -> Switch1/1
  Switch1/1 -> Delay One Step4/1, Triggered Subsystem3/1(In1)
  Add5/1 -> Switch1/3
  Switch Case3/3 -> Switch Case Action Subsystem17/Action
  Delay One Step4/1 -> If1/1, Add5/2
  Add4/1 -> Triggered Subsystem2/1(Inport), Triggered Subsystem3/2(Inport)
  Hall_U_Digital1/1 -> Mux/3
  Data Store Read3/1 -> Display7/1
  Combinatorial Logic/1 -> Cast To Single/1
  Hall_W_Digital1/1 -> Mux/2
  Switch Case Action Subsystem16/1(Out1) -> Add4/2
  Switch Case3/2 -> Switch Case Action Subsystem16/Action
  Switch Case Action Subsystem15/1(Out1) -> Add4/1
  Subtract1/1 -> Compare To Zero1/1, Switch Case Action Subsystem17/1(Inport), Switch Case3/1
  Compare To Zero1/1 -> Triggered Subsystem2/Trigger, Triggered Subsystem3/Trigger, Switch1/2
  Switch Case Action Subsystem17/1(Out1) -> Add4/3
  Hall_V_Digital1/1 -> Mux/1
  Mux/1 -> Combinatorial Logic/1
  Cast To Single/1 -> Delay One Step3/1, Subtract1/1

== system hall_effect_pos_vel_track/Function-Call Subsystem/If Action Subsystem1 ==
  Action Port : ActionPort  InitializeStates=reset  ActionPortLabel=if(u1 > 1000)
  Constant : Constant  Value=0  OutDataTypeStr=single  SampleTime=-1
  Data Store Write8 : DataStoreWrite  DataStoreName=MOT_VEL  IndexOptions=Index vector (dialog)  Indices=1  OutputSizes=1
  wires:
  Constant/1 -> Data Store Write8/1

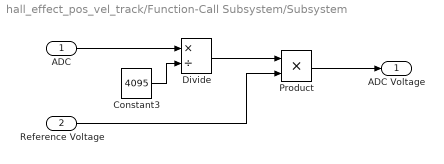
== system hall_effect_pos_vel_track/Function-Call Subsystem/Subsystem ==
  ADC : Inport
  Reference Voltage : Inport  Port=2
  Constant3 : Constant  Value=4095  OutDataTypeStr=single
  Divide : Product  Inputs=*/  OutDataTypeStr=single  RndMeth=Zero  SaturateOnIntegerOverflow=on
  Product : Product
  ADC Voltage : Outport
  wires:
  Divide/1 -> Product/1
  Constant3/1 -> Divide/2
  ADC/1 -> Divide/1
  Reference Voltage/1 -> Product/2
  Product/1 -> ADC Voltage/1

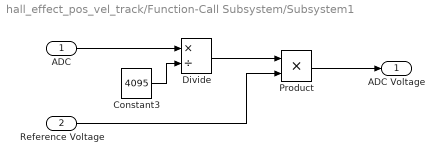
== system hall_effect_pos_vel_track/Function-Call Subsystem/Subsystem1 ==
  ADC : Inport
  Reference Voltage : Inport  Port=2
  Constant3 : Constant  Value=4095  OutDataTypeStr=single
  Divide : Product  Inputs=*/  OutDataTypeStr=single  RndMeth=Zero  SaturateOnIntegerOverflow=on
  Product : Product
  ADC Voltage : Outport
  wires:
  Product/1 -> ADC Voltage/1
  Reference Voltage/1 -> Product/2
  ADC/1 -> Divide/1
  Constant3/1 -> Divide/2
  Divide/1 -> Product/1

== system hall_effect_pos_vel_track/Function-Call Subsystem/Subsystem10 ==
  ADC : Inport
  Reference Voltage : Inport  Port=2
  Constant3 : Constant  Value=4095  OutDataTypeStr=single
  Divide : Product  Inputs=*/  OutDataTypeStr=single  RndMeth=Zero  SaturateOnIntegerOverflow=on
  Product : Product
  ADC Voltage : Outport
  wires:
  Divide/1 -> Product/1
  Constant3/1 -> Divide/2
  ADC/1 -> Divide/1
  Reference Voltage/1 -> Product/2
  Product/1 -> ADC Voltage/1

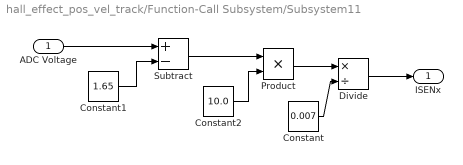
== system hall_effect_pos_vel_track/Function-Call Subsystem/Subsystem11 ==
  ADC Voltage : Inport
  Constant : Constant  Value=0.007  OutDataTypeStr=single
  Constant1 : Constant  Value=1.65  OutDataTypeStr=single
  Constant2 : Constant  Value=10.0  OutDataTypeStr=single
  Divide : Product  Inputs=*/
  Product : Product
  Subtract : Sum  Inputs=+-  OutDataTypeStr=single
  ISENx : Outport
  wires:
  Constant1/1 -> Subtract/2
  Constant2/1 -> Product/2
  Subtract/1 -> Product/1
  ADC Voltage/1 -> Subtract/1
  Product/1 -> Divide/1
  Constant/1 -> Divide/2
  Divide/1 -> ISENx/1

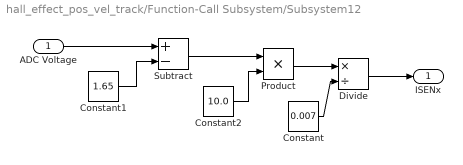
== system hall_effect_pos_vel_track/Function-Call Subsystem/Subsystem12 ==
  ADC Voltage : Inport
  Constant : Constant  Value=0.007  OutDataTypeStr=single
  Constant1 : Constant  Value=1.65  OutDataTypeStr=single
  Constant2 : Constant  Value=10.0  OutDataTypeStr=single
  Divide : Product  Inputs=*/
  Product : Product
  Subtract : Sum  Inputs=+-  OutDataTypeStr=single
  ISENx : Outport
  wires:
  Constant1/1 -> Subtract/2
  Constant2/1 -> Product/2
  Subtract/1 -> Product/1
  ADC Voltage/1 -> Subtract/1
  Product/1 -> Divide/1
  Constant/1 -> Divide/2
  Divide/1 -> ISENx/1

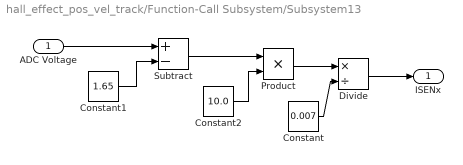
== system hall_effect_pos_vel_track/Function-Call Subsystem/Subsystem13 ==
  ADC Voltage : Inport
  Constant : Constant  Value=0.007  OutDataTypeStr=single
  Constant1 : Constant  Value=1.65  OutDataTypeStr=single
  Constant2 : Constant  Value=10.0  OutDataTypeStr=single
  Divide : Product  Inputs=*/
  Product : Product
  Subtract : Sum  Inputs=+-  OutDataTypeStr=single
  ISENx : Outport
  wires:
  Constant1/1 -> Subtract/2
  Constant2/1 -> Product/2
  Subtract/1 -> Product/1
  ADC Voltage/1 -> Subtract/1
  Product/1 -> Divide/1
  Constant/1 -> Divide/2
  Divide/1 -> ISENx/1

== system hall_effect_pos_vel_track/Function-Call Subsystem/Subsystem2 ==
  ADC : Inport
  Reference Voltage : Inport  Port=2
  Constant3 : Constant  Value=4095  OutDataTypeStr=single
  Divide : Product  Inputs=*/  OutDataTypeStr=single  RndMeth=Zero  SaturateOnIntegerOverflow=on
  Product : Product
  ADC Voltage : Outport
  wires:
  Divide/1 -> Product/1
  Constant3/1 -> Divide/2
  ADC/1 -> Divide/1
  Reference Voltage/1 -> Product/2
  Product/1 -> ADC Voltage/1

== system hall_effect_pos_vel_track/Function-Call Subsystem/Subsystem3 ==
  ADC Voltage : Inport
  Constant1 : Constant  Value=4.99  OutDataTypeStr=single
  Constant2 : Constant  Value=66.99  OutDataTypeStr=single
  Divide : Product  Inputs=*/  OutDataTypeStr=single  RndMeth=Zero  SaturateOnIntegerOverflow=on
  Product : Product
  VSENx : Outport
  wires:
  Constant1/1 -> Divide/2
  Constant2/1 -> Product/2
  Divide/1 -> Product/1
  Product/1 -> VSENx/1
  ADC Voltage/1 -> Divide/1

== system hall_effect_pos_vel_track/Function-Call Subsystem/Subsystem4 ==
  ADC Voltage : Inport
  Constant1 : Constant  Value=4.99  OutDataTypeStr=single
  Constant2 : Constant  Value=66.99  OutDataTypeStr=single
  Divide : Product  Inputs=*/  OutDataTypeStr=single  RndMeth=Zero  SaturateOnIntegerOverflow=on
  Product : Product
  VSENx : Outport
  wires:
  ADC Voltage/1 -> Divide/1
  Product/1 -> VSENx/1
  Divide/1 -> Product/1
  Constant2/1 -> Product/2
  Constant1/1 -> Divide/2

== system hall_effect_pos_vel_track/Function-Call Subsystem/Subsystem5 ==
  ADC Voltage : Inport
  Constant1 : Constant  Value=4.99  OutDataTypeStr=single
  Constant2 : Constant  Value=66.99  OutDataTypeStr=single
  Divide : Product  Inputs=*/  OutDataTypeStr=single  RndMeth=Zero  SaturateOnIntegerOverflow=on
  Product : Product
  VSENx : Outport
  wires:
  Constant1/1 -> Divide/2
  Constant2/1 -> Product/2
  Divide/1 -> Product/1
  Product/1 -> VSENx/1
  ADC Voltage/1 -> Divide/1

== system hall_effect_pos_vel_track/Function-Call Subsystem/Subsystem6 ==
  ADC : Inport
  Reference Voltage : Inport  Port=2
  Constant3 : Constant  Value=4095  OutDataTypeStr=single
  Divide : Product  Inputs=*/  OutDataTypeStr=single  RndMeth=Zero  SaturateOnIntegerOverflow=on
  Product : Product
  ADC Voltage : Outport
  wires:
  Divide/1 -> Product/1
  Constant3/1 -> Divide/2
  ADC/1 -> Divide/1
  Reference Voltage/1 -> Product/2
  Product/1 -> ADC Voltage/1

== system hall_effect_pos_vel_track/Function-Call Subsystem/Subsystem7 ==
  ADC Voltage : Inport
  Constant1 : Constant  Value=4.99  OutDataTypeStr=single
  Constant2 : Constant  Value=66.99  OutDataTypeStr=single
  Divide : Product  Inputs=*/  OutDataTypeStr=single  RndMeth=Zero  SaturateOnIntegerOverflow=on
  Product : Product
  VSENx : Outport
  wires:
  Constant1/1 -> Divide/2
  Constant2/1 -> Product/2
  Divide/1 -> Product/1
  Product/1 -> VSENx/1
  ADC Voltage/1 -> Divide/1

== system hall_effect_pos_vel_track/Function-Call Subsystem/Subsystem8 ==
  ADC : Inport
  Reference Voltage : Inport  Port=2
  Constant3 : Constant  Value=4095  OutDataTypeStr=single
  Divide : Product  Inputs=*/  OutDataTypeStr=single  RndMeth=Zero  SaturateOnIntegerOverflow=on
  Product : Product
  ADC Voltage : Outport
  wires:
  Divide/1 -> Product/1
  Constant3/1 -> Divide/2
  ADC/1 -> Divide/1
  Reference Voltage/1 -> Product/2
  Product/1 -> ADC Voltage/1

== system hall_effect_pos_vel_track/Function-Call Subsystem/Subsystem9 ==
  ADC : Inport
  Reference Voltage : Inport  Port=2
  Constant3 : Constant  Value=4095  OutDataTypeStr=single
  Divide : Product  Inputs=*/  OutDataTypeStr=single  RndMeth=Zero  SaturateOnIntegerOverflow=on
  Product : Product
  ADC Voltage : Outport
  wires:
  Divide/1 -> Product/1
  Constant3/1 -> Divide/2
  ADC/1 -> Divide/1
  Reference Voltage/1 -> Product/2
  Product/1 -> ADC Voltage/1

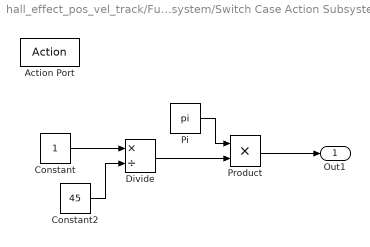
== system hall_effect_pos_vel_track/Function-Call Subsystem/Switch Case Action Subsystem15 ==
  Action Port : ActionPort  ActionPortLabel=case [ -5 ]:
  Constant : Constant  OutDataTypeStr=single
  Constant2 : Constant  Value=45  OutDataTypeStr=single
  Divide : Product  Inputs=*/  RndMeth=Zero  SaturateOnIntegerOverflow=on
  Pi : Constant  Value=pi  OutDataTypeStr=single
  Product : Product
  Out1 : Outport  OutputWhenDisabled=reset  InitialOutput=0
  wires:
  Product/1 -> Out1/1
  Constant2/1 -> Divide/2
  Divide/1 -> Product/2
  Constant/1 -> Divide/1
  Pi/1 -> Product/1

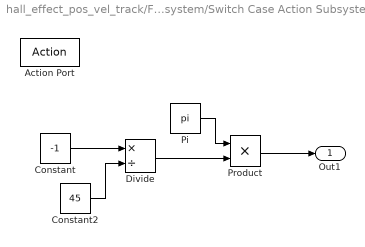
== system hall_effect_pos_vel_track/Function-Call Subsystem/Switch Case Action Subsystem16 ==
  Action Port : ActionPort  ActionPortLabel=case [ 5 ]:
  Constant : Constant  Value=-1  OutDataTypeStr=single
  Constant2 : Constant  Value=45  OutDataTypeStr=single
  Divide : Product  Inputs=*/  RndMeth=Zero  SaturateOnIntegerOverflow=on
  Pi : Constant  Value=pi  OutDataTypeStr=single
  Product : Product
  Out1 : Outport  OutputWhenDisabled=reset  InitialOutput=0
  wires:
  Product/1 -> Out1/1
  Constant2/1 -> Divide/2
  Divide/1 -> Product/2
  Constant/1 -> Divide/1
  Pi/1 -> Product/1

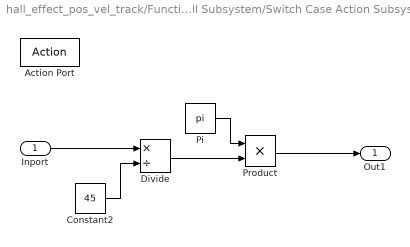
== system hall_effect_pos_vel_track/Function-Call Subsystem/Switch Case Action Subsystem17 ==
  Inport : Inport
  Action Port : ActionPort  ActionPortLabel=default:
  Constant2 : Constant  Value=45  OutDataTypeStr=single
  Divide : Product  Inputs=*/  RndMeth=Zero  SaturateOnIntegerOverflow=on
  Pi : Constant  Value=pi  OutDataTypeStr=single
  Product : Product
  Out1 : Outport  OutputWhenDisabled=reset  InitialOutput=0
  wires:
  Product/1 -> Out1/1
  Constant2/1 -> Divide/2
  Divide/1 -> Product/2
  Inport/1 -> Divide/1
  Pi/1 -> Product/1

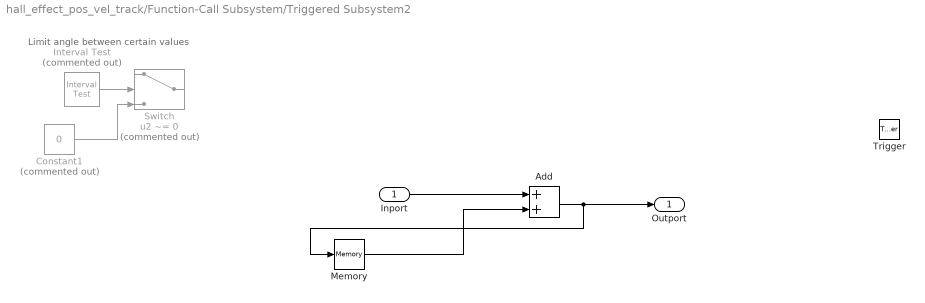
== system hall_effect_pos_vel_track/Function-Call Subsystem/Triggered Subsystem2 ==
  note: Limit angle between certain values
  Inport : Inport  OutDataTypeStr=single
  Trigger : TriggerPort  VariantControl=(inherit)
  Add : Sum
  Constant1 : Constant  Commented=on  Value=0  OutDataTypeStr=single
  Interval Test : simulink/Logic and Bit Operations/Interval Test  Commented=on  IntervalClosedRight=off  uplimit=2*pi  IntervalClosedLeft=off  lowlimit=0  OutDataTypeStr=boolean
  Memory : Memory  InheritSampleTime=on
  Switch : Switch  Commented=on  Criteria=u2 ~= 0  Threshold=90  OutDataTypeStr=single  SaturateOnIntegerOverflow=off  InputSameDT=off
  Outport : Outport  InitialOutput=0
  wires:
  Add/1 -> Outport/1, Memory/1
  Memory/1 -> Add/2
  Interval Test/1 -> Switch/2
  Constant1/1 -> Switch/3
  Inport/1 -> Add/1

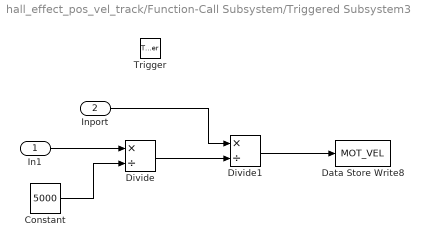
== system hall_effect_pos_vel_track/Function-Call Subsystem/Triggered Subsystem3 ==
  In1 : Inport  LatchByDelayingOutsideSignal=on
  Inport : Inport  Port=2
  Trigger : TriggerPort  VariantControl=(inherit)
  Constant : Constant  Value=5000  OutDataTypeStr=single
  Data Store Write8 : DataStoreWrite  DataStoreName=MOT_VEL  IndexOptions=Index vector (dialog)  Indices=1  OutputSizes=1
  Divide : Product  Inputs=*/
  Divide1 : Product  Inputs=*/
  wires:
  In1/1 -> Divide/1
  Constant/1 -> Divide/2
  Divide/1 -> Divide1/2
  Inport/1 -> Divide1/1
  Divide1/1 -> Data Store Write8/1
